simulink model "Final_Project_Ball_Beam_ControllerModel"  (R2017b)
settings: Solver=VariableStepAuto  StartTime=0.0  StopTime=10.0  RelTol=1e-3
undefined symbols (not defined in the file): d, g, J, L, m, r
settings Model: Creator=green  LastModifiedBy=green
settings SolverCC: AlgebraicLoopSolver=LineSearch
settings DebuggingCC: ArtificialAlgebraicLoopMsg=none

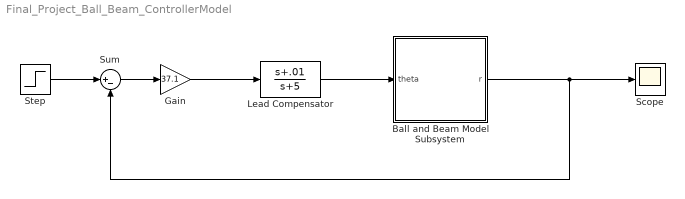
== system Final_Project_Ball_Beam_ControllerModel ==
  Ball and Beam Model Subsystem : Subsystem  TreatAsAtomicUnit=on
  Gain : Gain  Gain=37.1
  Lead Compensator : TransferFcn  Numerator=[1,.01]  Denominator=[1,5 ]
  Scope : Scope
  Step : Step  Time=0  SampleTime=0
  Sum : Sum  Inputs=|+-
  wires:
  Lead Compensator/1 -> Ball and Beam Model Subsystem/1(theta)
  Gain/1 -> Lead Compensator/1
  Sum/1 -> Gain/1
  Step/1 -> Sum/1
  Ball and Beam Model Subsystem/1(r) -> Scope/1, Sum/2

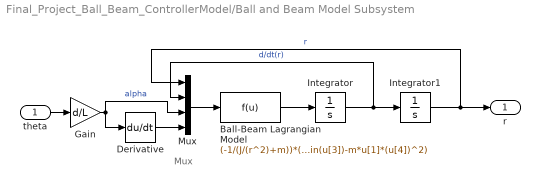
== system Final_Project_Ball_Beam_ControllerModel/Ball and Beam Model Subsystem ==
  note: Mux
  theta : Inport
  Ball-Beam Lagrangian Model : Fcn  Expr=(-1/(J/(r^2)+m))*(m*g*sin(u[3])-m*u[1]*(u[4])^2)
  Derivative : Derivative
  Gain : Gain  Gain=d/L
  Integrator : Integrator
  Integrator1 : Integrator
  Mux : Mux
  r : Outport
  wires:
  Integrator1/1 -> Mux/1, r/1  "r"
  Gain/1 -> Derivative/1, Mux/3  "alpha"
  Ball-Beam Lagrangian Model/1 -> Integrator/1
  Derivative/1 -> Mux/4
  Integrator/1 -> Mux/2, Integrator1/1  "d/dt(r)"
  Mux/1 -> Ball-Beam Lagrangian Model/1
  theta/1 -> Gain/1
